simulink model "modulacionFSK"  (R2019a)
settings: Solver=VariableStepAuto  StartTime=0.0  StopTime=10.0  RelTol=1e-3
settings Model: Creator=JORGE  LastModifiedBy=JORGE

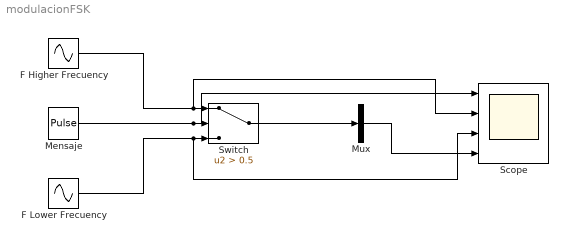
== system modulacionFSK ==
  F Higher Frecuency : Sin  Frequency=50  SampleTime=0.01
  F Lower Frecuency : Sin  Frequency=10  SampleTime=0.01
  Mensaje : DiscretePulseGenerator  PulseType=Time based  PulseWidth=50
  Mux : Mux  Inputs=1
  "Scope " : Scope  NumInputPorts=4
  "Switch " : Switch  Criteria=u2 > Threshold  Threshold=0.5
  wires:
  F Higher Frecuency/1 -> "Scope "/2, "Switch "/1
  Mensaje/1 -> "Scope "/1, "Switch "/2
  F Lower Frecuency/1 -> "Scope "/3, "Switch "/3
  "Switch "/1 -> Mux/1
  Mux/1 -> "Scope "/4
